simulink model "test"  (R2023b)
settings: Solver=VariableStepAuto  StartTime=0.0  StopTime=10.0  RelTol=1e-3
settings Model: Creator=trucd  LastModifiedBy=trucd

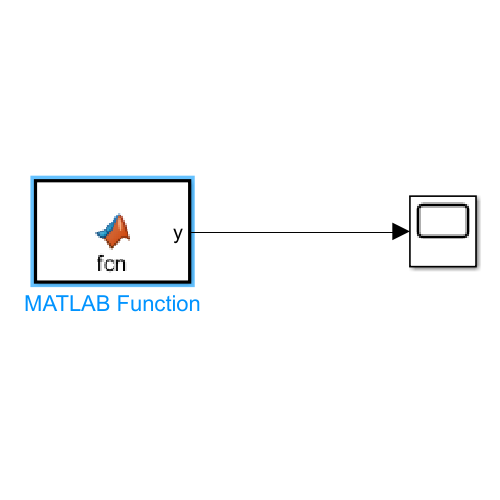
[thumbnail: Simulink's stored preview of the top-level diagram]
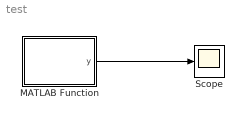
== system test ==
  MATLAB Function : MATLAB Function  TreatAsAtomicUnit=on
  Scope : Scope
  wires:
  MATLAB Function/1(y) -> Scope/1

== matlab function test/MATLAB Function ==
  data: y output
function y = fcn()
    clientID = "23265948";
    userName = "AQ0TNxAEGzkpKTozGS0fGxU";
    password = "DqS9WTqaYj0OawJhVw28n/0M";
y =5;
